simulink model "test_model"  (R2020b)
settings: Solver=FixedStepAuto  StartTime=0.0  StopTime=inf  RelTol=1e-3
libraries: DSX_Lib x8
settings Model: PacingRate=0.450000  Creator=16047  LastModifiedBy=16047

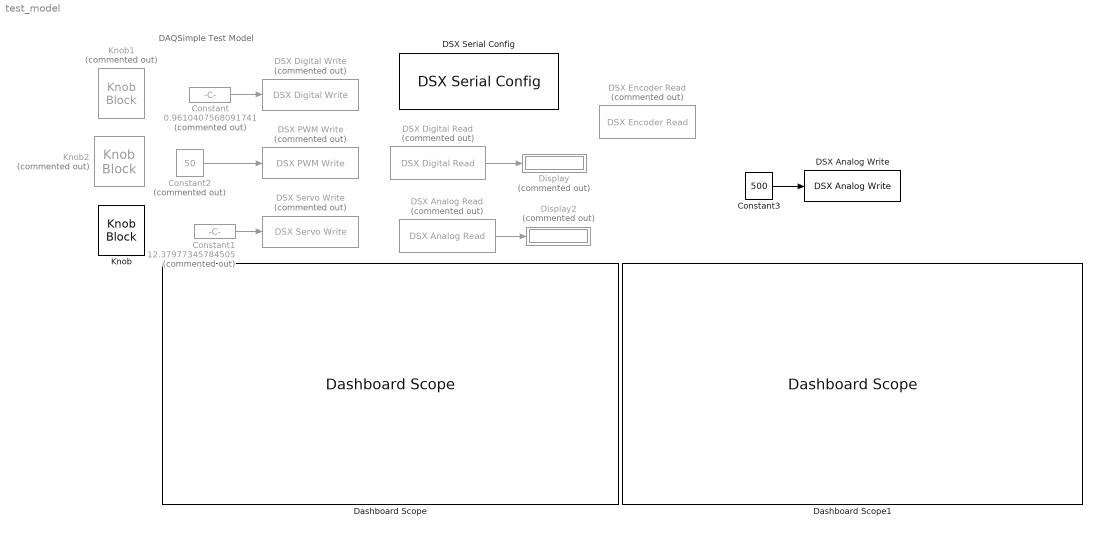
== system test_model ==
  note: DAQSimple Test Model
  Constant : Constant  Commented=on  Value=0.9610407568091741
  Constant1 : Constant  Commented=on  Value=12.37977345784505
  Constant2 : Constant  Commented=on  Value=50
  Constant3 : Constant  Value=500
  DSX Analog Read : DSX_Lib/DSX Blocks/DSX Analog Read  Commented=on  aread_pin=A0
      settings: SourceProductName=DSX Library
  DSX Analog Write : DSX_Lib/DSX Blocks/DSX Analog Write  analog_pin=DAC
      settings: SourceProductName=DSX Library
  DSX Digital Read : DSX_Lib/DSX Blocks/DSX Digital Read  Commented=on  read_pin=7
      settings: SourceProductName=DSX Library
  DSX Digital Write : DSX_Lib/DSX Blocks/DSX Digital Write  Commented=on  gpio_pin=9
      settings: SourceProductName=DSX Library
  DSX Encoder Read : DSX_Lib/DSX Blocks/DSX Encoder Read  Commented=on  eread_pin=2
      settings: SourceProductName=DSX Library
  DSX PWM Write : DSX_Lib/DSX Blocks/DSX PWM Write  Commented=on  pwm_pin=3  pwm_freq=980
      settings: SourceProductName=DSX Library
  DSX Serial Config : DSX_Lib/DSX Blocks/DSX Serial Config  BaudRate=9600
      settings: SourceProductName=DSX Library
  DSX Servo Write : DSX_Lib/DSX Blocks/DSX Servo Write  Commented=on  servo_pin=6
      settings: SourceProductName=DSX Library
  Dashboard Scope : DashboardScope  Ymin=-0.5  Ymax=1.5
  Dashboard Scope1 : DashboardScope  Ymin=0  Ymax=1024
  Display : Display  Commented=on
  Display2 : Display  Commented=on
  Knob : KnobBlock  ScaleMax=50
  Knob1 : KnobBlock  Commented=on  ScaleMax=1
  Knob2 : KnobBlock  Commented=on
  wires:
  Constant/1 -> DSX Digital Write/1
  DSX Analog Read/1 -> Display2/1
  Constant1/1 -> DSX Servo Write/1
  DSX Digital Read/1 -> Display/1
  Constant2/1 -> DSX PWM Write/1
  Constant3/1 -> DSX Analog Write/1
